simulink model "lab5accel"  (R2018b)
settings: Solver=FixedStepAuto  StartTime=0.0  StopTime=count  FixedStep=1  RelTol=1e-3
libraries: dspsrcs4 x2
settings Model: Creator=dfoster  LastModifiedBy=pete404
settings SFSimCC: SimUseLocalCustomCode=off
settings RTWCC: RTWUseLocalCustomCode=off
settings CodeAppCC: StateflowObjectComments=on

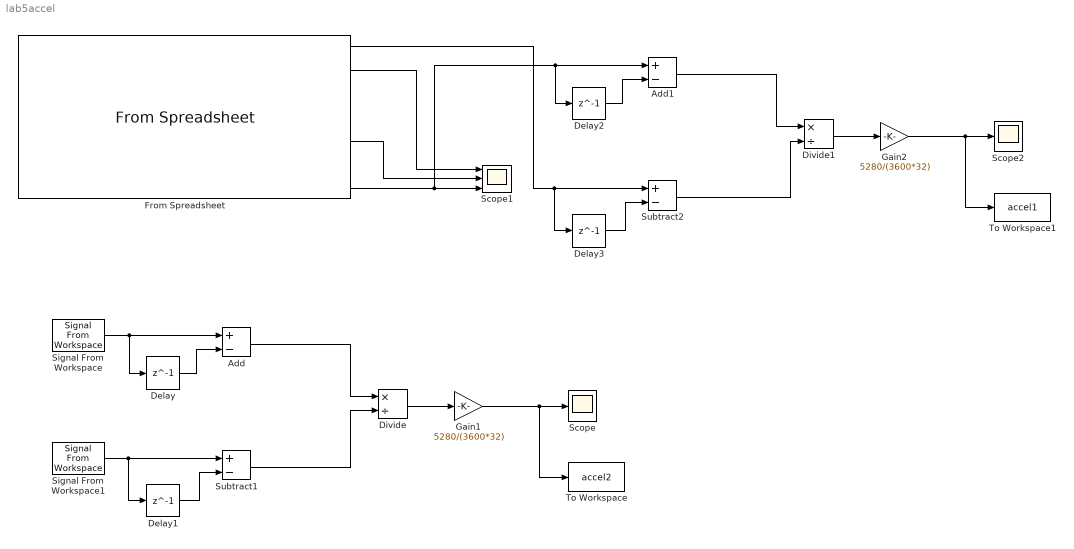
== system lab5accel ==
  Add : Sum  Inputs=+-
  Add1 : Sum  Inputs=+-
  Delay{,1..3} (4 alike) : Delay  DelayLength=1
  Divide : Product  Inputs=*/
  Divide1 : Product  Inputs=*/
  From Spreadsheet : FromSpreadsheet  FileName=datalog1.xlsx  SheetName=datalog1
  Gain1 : Gain  Gain=5280/(3600*32)
  Gain2 : Gain  Gain=5280/(3600*32)
  Scope : Scope
  Scope1 : Scope  NumInputPorts=3
  Scope2 : Scope
  Signal From Workspace : dspsrcs4/Signal From Workspace  X=speeds  Ts=1  nsamps=1  OutputAfterFinalValue=Setting to zero  ignoreOrWarnInputAndFrameLengths=off  OutputFrames=off
  Signal From Workspace1 : dspsrcs4/Signal From Workspace  X=times  Ts=1  nsamps=1  OutputAfterFinalValue=Setting to zero  ignoreOrWarnInputAndFrameLengths=off  OutputFrames=off
  Subtract1 : Sum  Inputs=+-
  Subtract2 : Sum  Inputs=+-
  To Workspace : ToWorkspace  VariableName=accel2  SampleTime=-1
      settings: Save2DSignal=2-D array (concatenate along first dimension)
  To Workspace1 : ToWorkspace  VariableName=accel1  SampleTime=-1
      settings: Save2DSignal=2-D array (concatenate along first dimension)
  wires:
  Delay/1 -> Add/2
  Signal From Workspace1/1 -> Delay1/1, Subtract1/1
  Delay1/1 -> Subtract1/2
  Add/1 -> Divide/1
  Subtract1/1 -> Divide/2
  Divide/1 -> Gain1/1
  Gain1/1 -> To Workspace/1, Scope/1
  From Spreadsheet/2 -> Scope1/1
  From Spreadsheet/5 -> Scope1/2
  Signal From Workspace/1 -> Delay/1, Add/1
  Delay2/1 -> Add1/2
  From Spreadsheet/1 -> Delay3/1, Subtract2/1
  Delay3/1 -> Subtract2/2
  Add1/1 -> Divide1/1
  Subtract2/1 -> Divide1/2
  Divide1/1 -> Gain2/1
  Gain2/1 -> To Workspace1/1, Scope2/1
  From Spreadsheet/7 -> Delay2/1, Add1/1, Scope1/3
